simulink model "controller_velocity_down"  (R2020a)
settings: Solver=FixedStepAuto  StartTime=0.0  StopTime=10.0  FixedStep=1/sim_freq  RelTol=1e-3
undefined symbols (not defined in the file): DiscIntNeverNeededParam, G_VD_OL_DENOM, G_VD_OL_NUM, K_wd, K_wi, K_wp, max_vel_z_down, max_vel_z_up, q_int_lim, vel_dterm_cutoff, vel_filt_denom, vel_filt_num
libraries: simulink x2
settings Model: Creator=francois  LastModifiedBy=murray

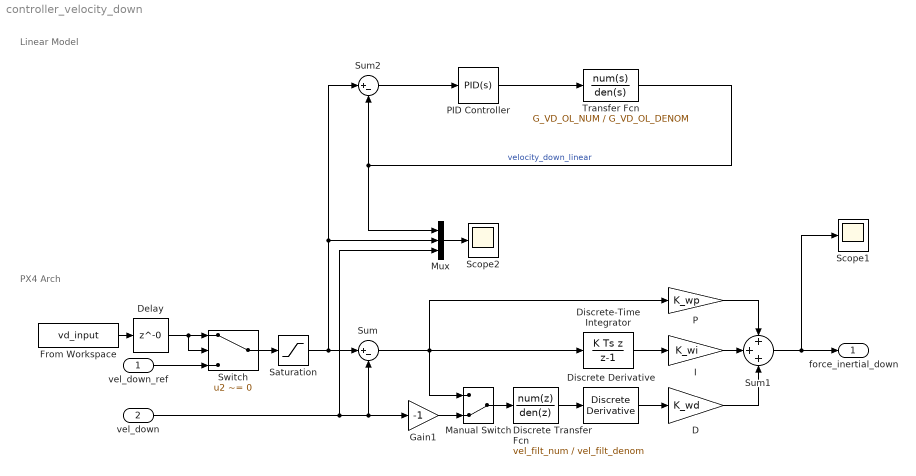
== system controller_velocity_down ==
  note: Linear Model
  note: PX4 Arch
  vel_down_ref : Inport
  vel_down : Inport  Port=2
  D : Gain  Gain=K_wd
  Delay : Delay  DelayLength=0
  Discrete Transfer Fcn : DiscreteTransferFcn  Numerator=vel_filt_num  Denominator=vel_filt_denom
  Discrete Derivative : simulink/Discrete/Discrete Derivative  gainval=1  ICPrevScaledInput=0.0  OutMin=[]  OutMax=[]  OutDataType=fixdt(1, 16)  OutScaling=2^-10  DoSatur=off
  Discrete-Time Integrator : DiscreteIntegrator  IntegratorMethod=Integration: Backward Euler  gainval=1  SampleTime=-1  UpperSaturationLimit=q_int_lim  LowerSaturationLimit=-q_int_lim  ICPrevOutput=DiscIntNeverNeededParam  ICPrevScaledInput=DiscIntNeverNeededParam
  From Workspace : FromWorkspace  VariableName=vd_input
  Gain1 : Gain  Gain=-1
  I : Gain  Gain=K_wi
  Manual Switch : ManualSwitch  CurrentSetting=0
  Mux : Mux  Inputs=3
  P : Gain  Gain=K_wp
  PID Controller : simulink/Continuous/PID Controller  Controller=PID  Form=Parallel  TimeDomain=Continuous-time  UseExternalTs=off  SampleTime=-1  IntegratorMethod=Forward Euler  FilterMethod=Forward Euler  ControllerParametersSource=internal  P=K_wp  I=K_wi  D=K_wd  UseFilter=on  N=vel_dterm_cutoff*10  TunerSelectOption=Transfer Function Based (PID Tuner App)  InitialConditionSource=internal  InitialConditionForIntegrator=0  InitialConditionForFilter=0  DifferentiatorICPrevScaledInput=0  ExternalReset=none  TrackingMode=off  Kt=1  LimitOutput=off  UpperSaturationLimit=inf  LowerSaturationLimit=-inf  LinearizeAsGain=on  AntiWindupMode=none  Kb=1  POutMin=[]  POutMax=[]  IOutMin=[]  IOutMax=[]  DOutMin=[]  DOutMax=[]  NOutMin=[]  NOutMax=[]  SumOutMin=[]  SumOutMax=[]  SaturationOutMin=[]  SaturationOutMax=[]  PParamMin=[]  PParamMax=[]  IParamMin=[]  IParamMax=[]  DParamMin=[]  DParamMax=[]  NParamMin=[]  NParamMax=[]  KbParamMin=[]  KbParamMax=[]  KtParamMin=[]  KtParamMax=[]  KbOutMin=[]  KbOutMax=[]  KtOutMin=[]  KtOutMax=[]  IntegratorOutMin=[]  IntegratorOutMax=[]  FilterOutMin=[]  FilterOutMax=[]  SumI1OutMin=[]  SumI1OutMax=[]  SumI2OutMin=[]  SumI2OutMax=[]  SumI3OutMin=[]  SumI3OutMax=[]  SumI4OutMin=[]  SumI4OutMax=[]  SumDOutMin=[]  SumDOutMax=[]  DifferentiatorOutMin=[]  DifferentiatorOutMax=[]  FilterDiffOutCoefMin=[]  FilterDiffOutCoefMax=[]  ReciprocalOutMin=[]  ReciprocalOutMax=[]  SumDenOutMin=[]  SumDenOutMax=[]  SumNumOutMin=[]  SumNumOutMax=[]  DivideOutMin=[]  DivideOutMax=[]  UdiffTsProdOutMin=[]  UdiffTsProdOutMax=[]  NTsProdOutMin=[]  NTsProdOutMax=[]  UintegralTsProdOutMin=[]  UintegralTsProdOutMax=[]  UngainTsProdOutMin=[]  UngainTsProdOutMax=[]  IntegratorContinuousStateAttributes=''  IntegratorStateMustResolveToSignalObject=off  IntegratorRTWStateStorageClass=Auto  FilterContinuousStateAttributes=''  FilterStateMustResolveToSignalObject=off  FilterRTWStateStorageClass=Auto  ParallelPVariant=InternalParameters  IdealPVariant=Disabled  IVariant=InternalParameters  DVariant=InternalParameters  IntegratorVariant=Continuous  SatVariant=Disabled  AWVariant=Passthrough  PCopyVariant=Disabled  TRVariant=Disabled  FdbkBlocksVariant=Forward  IdealPFdbkVariant=Disabled  SatFdbkVariant=Disabled  DerivativeFilterVariant=ContFilter  NVariant=InternalParameters  NCopyVariant=Disabled  FilterICVariant=InternalICsFilter  IntegratorICVariant=InternalICs  ExternalResetVariant=Disabled  TRSumVariant=Passthrough  SumFdbkVariant=Disabled  SumVariant=Sum_PID  TsampFilterVariant=InternalTs  TsampNgainVariant=Passthrough  TsampIntegralVariant=Passthrough
  Saturation : Saturate  UpperLimit=max_vel_z_up  LowerLimit=max_vel_z_down
  Scope1 : Scope
  Scope2 : Scope
  Sum : Sum  Inputs=|+-
  Sum1 : Sum  Inputs=+++
  Sum2 : Sum  Inputs=|+-
  Switch : Switch  Criteria=u2 ~= 0
  Transfer Fcn : TransferFcn  Numerator=G_VD_OL_NUM  Denominator=G_VD_OL_DENOM
  force_inertial_down : Outport  VectorParamsAs1DForOutWhenUnconnected=off
  wires:
  Saturation/1 -> Sum/1, Mux/2, Sum2/1
  D/1 -> Sum1/3
  Transfer Fcn/1 -> Mux/1, Sum2/2  "velocity_down_linear"
  Manual Switch/1 -> Discrete Transfer Fcn/1
  From Workspace/1 -> Delay/1
  Sum/1 -> Discrete-Time Integrator/1, Manual Switch/1, P/1
  Sum1/1 -> Scope1/1, force_inertial_down/1
  I/1 -> Sum1/2
  Discrete-Time Integrator/1 -> I/1
  Discrete Derivative/1 -> D/1
  Gain1/1 -> Manual Switch/2
  Delay/1 -> Switch/2, Switch/1
  Discrete Transfer Fcn/1 -> Discrete Derivative/1
  vel_down_ref/1 -> Switch/3
  PID Controller/1 -> Transfer Fcn/1
  Switch/1 -> Saturation/1
  Sum2/1 -> PID Controller/1
  P/1 -> Sum1/1
  vel_down/1 -> Mux/3, Gain1/1, Sum/2
  Mux/1 -> Scope2/1
